simulink model "verify_Solar_Collector_basic_mdl"  (R2018b)
settings: Solver=ode45  StartTime=0.0  StopTime=24*3600  MaxStep=100  RelTol=1e-3  EnableMultiTasking=on
libraries: carnot x13, simulink x1
settings Model: Creator=drhf  LastModifiedBy=P41573
settings DataIOCC: LimitDataPoints=on  SaveFormat=Array  SignalLoggingSaveFormat=ModelDataLogs
settings OptimizationCC: ExpressionDepthLimit=2147483647  LifeSpan=inf
settings DebuggingCC: UnderspecifiedInitializationDetection=Classic  MergeDetectMultiDrivingBlocksExec=none  SolverPrmCheckMsg=warning  FcnCallInpInsideContextMsg=warning  StateNameClashWarn=warning  SFUnexpectedBacktrackingDiag=warning  SFNoUnconditionalDefaultTransitionDiag=warning  SFExecutionAtInitializationDiag=none
settings HardwareCC: ProdBitPerPointer=32  ProdBitPerSizeT=32  ProdBitPerPtrDiffT=32  ProdLargestAtomicFloat=None  ProdIntDivRoundTo=Undefined  ProdEndianess=Unspecified  ProdWordSize=32  ProdHWDeviceType=32-bit Generic
settings ModelReferenceCC: PropagateSignalLabelsOutOfModel=off
settings SFSimCC: SimUseLocalCustomCode=off
settings RTWCC: RTWUseLocalCustomCode=off
settings CodeAppCC: StateflowObjectComments=on
settings GRTTargetCC: TargetLangStandard=C89/C90 (ANSI)  GeneratePreprocessorConditionals=Disable all  CombineOutputUpdateFcns=off  GRTInterface=on
settings ConfigComp: CovMetricSettings=dw  CovHtmlReporting=on  CovSaveCumulativeToWorkspaceVar=on  CovSaveSingleToWorkspaceVar=on  CovExternalEMLEnable=off

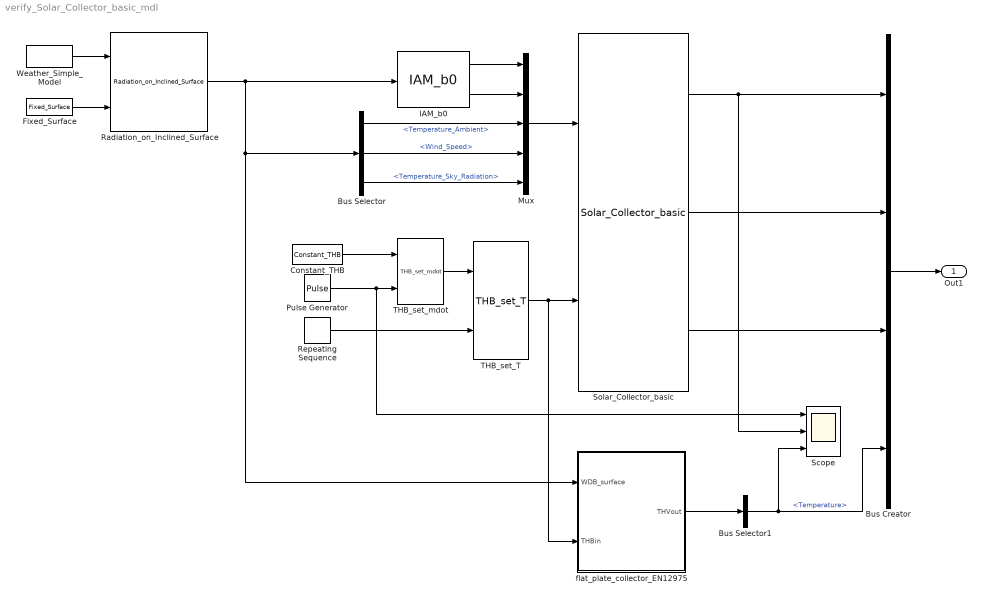
== system verify_Solar_Collector_basic_mdl ==
  Bus Creator : BusCreator  Inputs=4
  Bus Selector : BusSelector  OutputSignals=Temperature_Ambient,Wind_Speed,Temperature_Sky_Radiation
  Bus Selector1 : BusSelector  OutputSignals=Temperature
  Constant_THB : carnot/Source/Simple/Constant_THB  t=40  mdot=100/3600  p=1e5  mID=No Pressure Drop  fluid=Water  mix=0  mix2=0  mix3=0  dia=0.02  hgt=0
  Fixed_Surface : carnot/Weather/Fixed_Surface  colangle=30  colazi=0  colrot=0
  IAM_b0 : carnot/Source/Solar_Thermal/IncidenceAngleModifier/IAM_b0  fta=0.8  b0=0.12  Kd=0.92
  Mux : Mux  Inputs=5
  Pulse Generator : DiscretePulseGenerator  PulseType=Time based  Amplitude=100/3600  Period=7*3600  PulseWidth=50
  Radiation_on_Inclined_Surface : carnot/Weather/Radiation_on_Inclined_Surface  sky=Perez 1990  reflect=0.2
  Repeating Sequence : simulink/Sources/Repeating Sequence  rep_seq_t=[0 7 7.1 14 14.1 21 21.1 24]*3600  rep_seq_y=[65 65 75 75 85 85 95 95]
  Scope : Scope  NumInputPorts=3
  Solar_Collector_basic : carnot/Basic/Thermal_Models/Solar_Collector_basic  acol=2.5  c1=3.757  c2=0.0147  c3=0  c4=0  c5=7062  c6=0  tini=20
  THB_set_T : carnot/Source/Simple/THB_set_T
  THB_set_mdot : carnot/Source/Simple/THB_set_mdot
  Weather_Simple_Model : carnot/Weather/Weather_Simple_Model  lat=60  Ibn=900  Idg=100  tamb=5  deltaTsky=-6  rh=50  precip="10e-3/24/3600           % 10 mm in 24 h"  cloud=0.125  p=1013e2  vw=1  wdir=270
  flat_plate_collector_EN12975 : Subsystem  mask(collector){acol=2.5, fta=0.8, c1=3.757, c2=0.0147, c3=0, c4=0, c5=7062, c6=0, b0=0.12, Kd=0.92, len=2.3, tini=20}
      mask prompts: acol "A : collector surface  [m²]"; fta "F'(TauAlfa) : collector efficiency factor x effective transmittance-absorptance product for direct solar radiation at normal incidence"; c1 "c1 : heat loss coefficient at (Tm-Ta)=0  [W/(m²*K)]"; c2 "c2: temperature dependence of the heat loss coefficient [W/(m*K)²]"; c3 "c3 : wind speed dependence of the heat loss coefficient [J/(m³K)]"; c4 "c4 : sky temperature dependence of the heat loss coefficient [W/(m²K)]"; c5 "c5 : effective thermal capacity [J/(m²K)]"; c6 "c6 : wind dependence in the zero loss efficiency [s/m]"; b0 "b0 : constant for the calculation of the incident angle modifier (direct radiation)"; Kd "Kd : Incidence angle modifier diffuse radiation"; len "length between inlet and outlet [m]"; tini "initial temperature [degree centigrade]"
      mask help:
      | Collector model according to EN 12975 standard.
      | Energy balance:
      | mdot cp (Tout-Tin) /A = F'(TauAlfa) Kdir Idir + F'(TauAlfa) Kdfu Idfu
      |        - c1 (Tm-Tamb) - c2 (Tm-Tamb)^2 - c3 v_wind (Tm-Ta) - c6 v_wind Iglb
      |        + c4 (ELongwave - sigmaSB*(Tamb+273.15)^4) - c5 dTm/dt
      |
      | Often in test reports the optical efficiency or conversion factor eta0 is given.
      | The correlation for F'(TauAlfa) is:
      | eta0 = F'(TauAlfa) * (Kdir(15°)*0.85 + Kdfu*0.15)
      | or
      | F'(TauAlfa) = eta0 / (Kdir(15°)*0.85 + Kdfu*0.15)
      mask init:
      | acol = max(acol, 0.01);
      | c5 = max(c5, 0.001);
      mask Help: eval('htmlhelp (''chap_4_2c.htm#collector_flat_plate'')')
      mask Display: disp('solar thermal\nflat plate\ncollector\nEN 12975')
  Out1 : Outport
  wires:
  Constant_THB/1 -> THB_set_mdot/1
  Pulse Generator/1 -> Scope/1, THB_set_mdot/2
  Bus Creator/1 -> Out1/1
  THB_set_T/1 -> flat_plate_collector_EN12975/2(THBin), Solar_Collector_basic/2
  THB_set_mdot/1 -> THB_set_T/1
  Repeating Sequence/1 -> THB_set_T/2
  Solar_Collector_basic/2 -> Bus Creator/2
  Solar_Collector_basic/1 -> Scope/2, Bus Creator/1
  Solar_Collector_basic/3 -> Bus Creator/3
  Fixed_Surface/1 -> Radiation_on_Inclined_Surface/2
  Weather_Simple_Model/1 -> Radiation_on_Inclined_Surface/1
  Radiation_on_Inclined_Surface/1 -> IAM_b0/1, Bus Selector/1, flat_plate_collector_EN12975/1(WDB_surface)
  IAM_b0/1 -> Mux/1
  IAM_b0/2 -> Mux/2
  Bus Selector/1 -> Mux/3  "<Temperature_Ambient>"
  Bus Selector/2 -> Mux/4  "<Wind_Speed>"
  Bus Selector/3 -> Mux/5  "<Temperature_Sky_Radiation>"
  Mux/1 -> Solar_Collector_basic/1
  flat_plate_collector_EN12975/1(THVout) -> Bus Selector1/1
  Bus Selector1/1 -> Scope/3, Bus Creator/4  "<Temperature>"

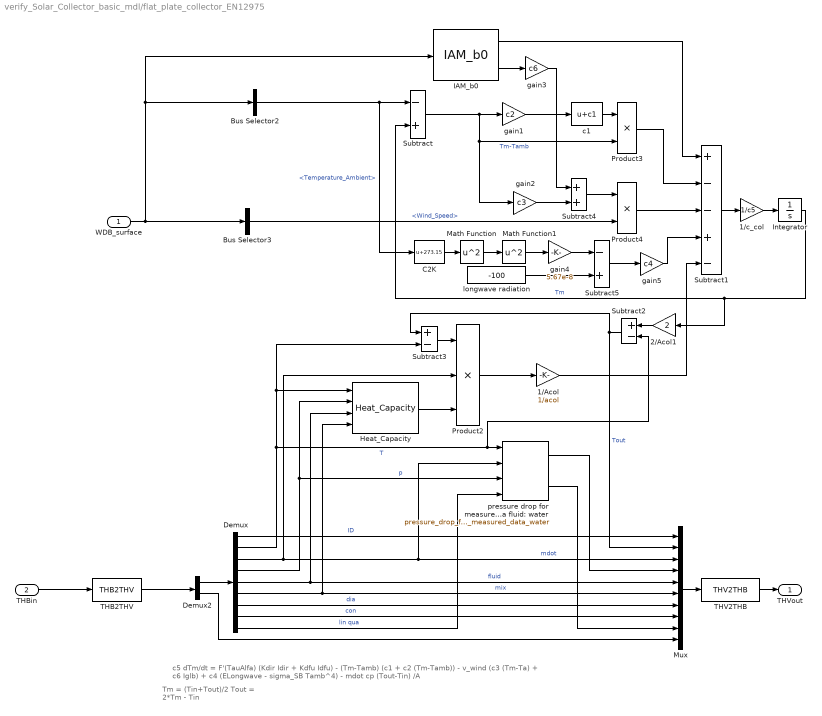
== system verify_Solar_Collector_basic_mdl/flat_plate_collector_EN12975 ==
  note: c5 dTm/dt = F'(TauAlfa) (Kdir Idir + Kdfu Idfu) - (Tm-Tamb) (c1 + c2 (Tm-Tamb)) - v_wind (c3 (Tm-Ta) + c6 Iglb) + c4 (ELongwave - sigma_SB Tamb^4) - mdot cp (Tout-Tin) /A
  note: Tm = (Tin+Tout)/2
      | Tout = 2*Tm - Tin
  WDB_surface : Inport
  THBin : Inport  Port=2
  1/Acol : Gain  Gain=1/acol
  1/c_col : Gain  Gain=1/c5
  2/Acol1 : Gain  Gain=2
  Bus Selector2 : BusSelector  OutputSignals=Temperature_Ambient
  Bus Selector3 : BusSelector  OutputSignals=Wind_Speed
  C2K : Bias  Bias=273.15
  Demux : Demux  Outputs=[1 1 1 1 1 1 1 1 2]
  Demux2 : Demux  Outputs=[10 -1]
  Heat_Capacity : carnot/Basic/Material_Properties/Heat_Capacity  VariantControl=CarlibClassic  INPUTARGUMENTS=state variables (classic)  DEBUGLEVEL=DEBUGLEVEL  MAXTOTALWARNINGS=inf  MAXCONSECUTIVEWARNINGS=inf  WRITETOFILE=0  FILENAME='errors.txt'
  IAM_b0 : carnot/Source/Solar_Thermal/IncidenceAngleModifier/IAM_b0  fta=fta  b0=b0  Kd=Kd
  Integrator : Integrator  InitialCondition=tini
  Math Function : Math  Operator=square  SaturateOnIntegerOverflow=on
  Math Function1 : Math  Operator=square  SaturateOnIntegerOverflow=on
  Mux : Mux  Inputs=10
  Product2 : Product  Inputs=3  RndMeth=Zero
  Product3 : Product  RndMeth=Zero
  Product4 : Product  RndMeth=Zero
  Subtract : Sum  Inputs=-+
  Subtract1 : Sum  Inputs=+--+-
  Subtract2 : Sum  Inputs=+-
  Subtract3 : Sum  Inputs=+-
  Subtract4 : Sum  Inputs=2
  Subtract5 : Sum  Inputs=-+
  THB2THV : carnot/Toolbox/THB2THV
  THV2THB : carnot/Toolbox/THV2THB
  c1 : Bias  Bias=c1
  gain1 : Gain  Gain=c2
  gain2 : Gain  Gain=c3
  gain3 : Gain  Gain=c6
  gain4 : Gain  Gain=5.67e-8
  gain5 : Gain  Gain=c4
  longwave radiation : Constant  Value=-100
  pressure drop for measured data fluid: water : carnot/Source/Solar_Thermal/PressureDropCollector/pressure_drop_for_measured_data_water  mdottest=0.01*1.96  ttest=20  pdroptest=158*1.96  aonecol=1.96  acol=acol
  THVout : Outport  InitialOutput=0
  wires:
  Demux/3 -> pressure drop for measured data fluid: water/2, Mux/3, Product2/2  "mdot"
  Demux/5 -> Heat_Capacity/3, Mux/5  "fluid"
  Demux/1 -> Mux/1  "ID"
  Demux2/1 -> Demux/1
  THBin/1 -> THB2THV/1
  Demux/4 -> Heat_Capacity/2, pressure drop for measured data fluid: water/3  "p"
  Demux/6 -> Heat_Capacity/4, Mux/6  "mix"
  pressure drop for measured data fluid: water/1 -> Mux/4
  pressure drop for measured data fluid: water/2 -> Mux/9
  Demux/9 -> pressure drop for measured data fluid: water/4  "lin qua"
  Demux/8 -> Mux/8  "con"
  Demux/7 -> Mux/7  "dia"
  Demux2/2 -> Mux/10
  Demux/2 -> Heat_Capacity/1, Subtract3/2, pressure drop for measured data fluid: water/1, Subtract2/2  "T"
  Bus Selector2/1 -> C2K/1, Subtract/1  "<Temperature_Ambient>"
  Subtract1/1 -> 1/c_col/1
  1/c_col/1 -> Integrator/1
  Heat_Capacity/1 -> Product2/3
  Product2/1 -> 1/Acol/1
  Integrator/1 -> 2/Acol1/1, Subtract/2  "Tm"
  Subtract3/1 -> Product2/1
  Subtract/1 -> gain1/1, Product3/2, gain2/1  "Tm-Tamb"
  IAM_b0/1 -> Subtract1/1
  gain1/1 -> c1/1
  c1/1 -> Product3/1
  Product3/1 -> Subtract1/2
  gain2/1 -> Subtract4/2
  IAM_b0/2 -> gain3/1
  gain3/1 -> Subtract4/1
  Product4/1 -> Subtract1/3
  Subtract4/1 -> Product4/1
  Bus Selector3/1 -> Product4/2  "<Wind_Speed>"
  Math Function/1 -> Math Function1/1
  C2K/1 -> Math Function/1
  Math Function1/1 -> gain4/1
  gain4/1 -> Subtract5/1
  longwave radiation/1 -> Subtract5/2
  1/Acol/1 -> Subtract1/5
  Subtract5/1 -> gain5/1
  gain5/1 -> Subtract1/4
  Subtract2/1 -> Mux/2, Subtract3/1  "Tout"
  2/Acol1/1 -> Subtract2/1
  THB2THV/1 -> Demux2/1
  THV2THB/1 -> THVout/1
  Mux/1 -> THV2THB/1
  WDB_surface/1 -> Bus Selector3/1, IAM_b0/1, Bus Selector2/1
